simulink model "simu_Juliana2024"  (R2023b)
settings: Solver=VariableStepAuto  StartTime=0.0  StopTime=Tsim  RelTol=1e-3
values from neighbouring files (symbols this model uses):
  ac = 9.6832*10^-4    (= 0.00096832)    [Juliana2024.m]
  ad = 0.9077    [Juliana2024.m]
  bc = -1.0482*10^-4    (= -0.00010482)    [Juliana2024.m]
  bd = -0.01    [Juliana2024.m]
  cond_inicial = 0    [Juliana2024.m]
  K1 = K*H1    [Juliana2024.m]
  K2 = K*H2    [Juliana2024.m]
  K3 = K*F1    [Juliana2024.m]
  ke = ke(1,:)    [Juliana2024.m]
  kr = sum(K)    [Juliana2024.m]
  m1c = 2.3090*10^-4    (= 0.0002309)    [Juliana2024.m]
  m1d = 0.022    [Juliana2024.m]
  m2c = 9.5293*10^-4    (= 0.00095293)    [Juliana2024.m]
  m2d = 0.0908    [Juliana2024.m]
  ref = ref-cond_inicial    (= 1)    [Juliana2024.m]
  s = tf('s')    [Juliana2024.m]
  Tref = 0    [Juliana2024.m]
  Ts = 100    [Juliana2024.m]
  Tsim = 100000    [Juliana2024.m]
  z = tf('z',Ts)    [Juliana2024.m]
undefined symbols (not defined in the file or in its folder): u_max, u_min, y_max, y_min
libraries: cstblocks x5
settings Model: Creator=junio  LastModifiedBy=sergio

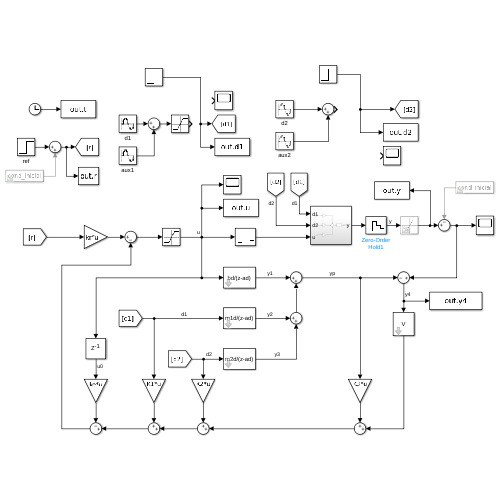
[thumbnail: Simulink's stored preview of the top-level diagram]
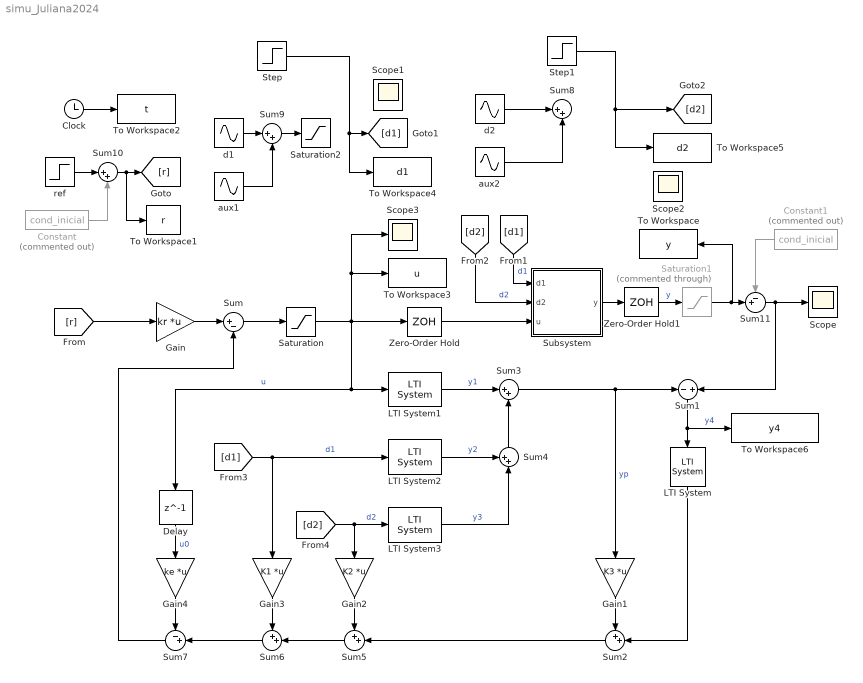
== system simu_Juliana2024 ==
  Clock : Clock
  Constant : Constant  Commented=on  Value=cond_inicial
  Constant1 : Constant  Commented=on  Value=cond_inicial
  Delay : Delay  DelayLength=1  SampleTime=Ts
  Gain : Gain  Gain=kr  Multiplication=Matrix(K*u)
  Gain1 : Gain  Gain=K3  Multiplication=Matrix(K*u)
  Gain2 : Gain  Gain=K2  Multiplication=Matrix(K*u)
  Gain3 : Gain  Gain=K1  Multiplication=Matrix(K*u)
  Gain4 : Gain  Gain=ke  Multiplication=Matrix(K*u)
  LTI System : cstblocks/LTI System  sys=V  IC=[]  PadeOrder=0
  LTI System1 : cstblocks/LTI System  sys=bd/(z-ad)  IC=[]  PadeOrder=0
  LTI System2 : cstblocks/LTI System  sys=m1d/(z-ad)  IC=[]  PadeOrder=0
  LTI System3 : cstblocks/LTI System  sys=m2d/(z-ad)  IC=[]  PadeOrder=0
  Saturation : Saturate  UpperLimit=u_max  LowerLimit=u_min
  Saturation1 : Saturate  Commented=through  UpperLimit=y_max  LowerLimit=y_min
  Saturation2 : Saturate  UpperLimit=80  LowerLimit=5
  Scope{,1..3} (4 alike) : Scope
  Step : Step  Time=30000  SampleTime=Ts
  Step1 : Step  Time=60000  After=0.5  SampleTime=Ts
  Subsystem : Subsystem
  Sum : Sum  Inputs=|+-
  Sum1 : Sum  Inputs=-|+
  Sum{3,8..10} (4 alike) : Sum  Inputs=|++
  Sum11 : Sum  Inputs=-+|
  Sum{2,4..6} (4 alike) : Sum  Inputs=++|
  Sum7 : Sum  Inputs=-+|
  To Workspace : ToWorkspace  VariableName=y  SampleTime=Ts
  To Workspace1 : ToWorkspace  VariableName=r  SampleTime=Ts
  To Workspace2 : ToWorkspace  VariableName=t  SampleTime=Ts
  To Workspace3 : ToWorkspace  VariableName=u  SampleTime=Ts
  To Workspace4 : ToWorkspace  VariableName=d1  SampleTime=Ts
  To Workspace5 : ToWorkspace  VariableName=d2  SampleTime=Ts
  To Workspace6 : ToWorkspace  VariableName=y4  SampleTime=Ts
  Zero-Order Hold : ZeroOrderHold  SampleTime=Ts
  Zero-Order Hold1 : ZeroOrderHold  SampleTime=Ts
  aux1 : Sin  Amplitude=0.5  Frequency=8*2*pi/Tsim  Phase=-pi/4  SampleTime=Ts
  aux2 : Sin  Amplitude=0.5  Frequency=8*2*pi/Tsim  Phase=-pi/1.25  SampleTime=Ts
  d1 : Sin  Amplitude=80  Frequency=2*pi/Tsim  Phase=-pi/4  SampleTime=Ts
  d2 : Sin  Amplitude=7.5  Bias=35.5  Frequency=2.25*pi/Tsim  Phase=-pi/1.25  SampleTime=Ts
  ref : Step  Time=Tref  After=ref  SampleTime=Ts
  wires:
  Gain/1 -> Sum/1
  Sum/1 -> Saturation/1
  Sum1/1 -> To Workspace6/1, LTI System/1  "y4"
  LTI System/1 -> Sum2/2
  LTI System1/1 -> Sum3/1  "y1"
  Sum3/1 -> Sum1/1, Gain1/1  "yp"
  Gain1/1 -> Sum2/1
  LTI System2/1 -> Sum4/1  "y2"
  LTI System3/1 -> Sum4/2  "y3"
  Sum4/1 -> Sum3/2
  [d1] -> Gain3/1, LTI System2/1  "d1"
  [d2] -> LTI System3/1, Gain2/1  "d2"
  Gain2/1 -> Sum5/1
  Sum2/1 -> Sum5/2
  Gain3/1 -> Sum6/1
  Sum5/1 -> Sum6/2
  Sum6/1 -> Sum7/2
  Gain4/1 -> Sum7/1
  Delay/1 -> Gain4/1  "u0"
  Sum7/1 -> Sum/2
  Saturation/1 -> To Workspace3/1, Scope3/1, Delay/1, LTI System1/1, Zero-Order Hold/1  "u"
  Clock/1 -> To Workspace2/1
  d2/1 -> Sum8/1
  aux2/1 -> Sum8/2
  d1/1 -> Sum9/1
  aux1/1 -> Sum9/2
  Zero-Order Hold1/1 -> Saturation1/1  "y"
  Constant1/1 -> Sum11/1
  Sum11/1 -> Sum1/2, Scope/1
  Sum10/1 -> To Workspace1/1, [r]
  ref/1 -> Sum10/1
  Constant/1 -> Sum10/2
  [r] -> Gain/1
  Sum9/1 -> Saturation2/1
  Subsystem/1(y) -> Zero-Order Hold1/1
  Zero-Order Hold/1 -> Subsystem/3(u)
  [d1] -> Subsystem/1(d1)  "d1"
  [d2] -> Subsystem/2(d2)  "d2"
  Step1/1 -> [d2], To Workspace5/1
  Step/1 -> To Workspace4/1, [d1]
  Saturation1/1 -> Sum11/2, To Workspace/1

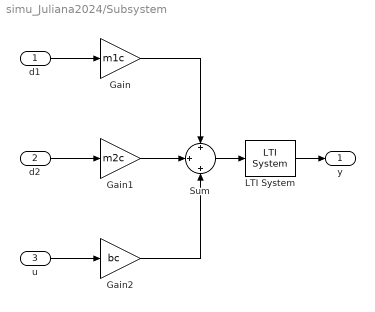
== system simu_Juliana2024/Subsystem ==
  d1 : Inport
  d2 : Inport  Port=2
  u : Inport  Port=3
  Gain : Gain  Gain=m1c
  Gain1 : Gain  Gain=m2c
  Gain2 : Gain  Gain=bc
  LTI System : cstblocks/LTI System  sys=1/(s+ac)  IC=[]  PadeOrder=0
  Sum : Sum  Inputs=+|+|+
  y : Outport
  wires:
  LTI System/1 -> y/1
  Sum/1 -> LTI System/1
  u/1 -> Gain2/1
  d2/1 -> Gain1/1
  d1/1 -> Gain/1
  Gain2/1 -> Sum/3
  Gain1/1 -> Sum/2
  Gain/1 -> Sum/1
